simulink model "GNC_exp_simulink_vision"  (R2018a)
settings: Solver=FixedStepAuto  StartTime=0.0  StopTime=50  FixedStep=0.2  MaxStep=0.5  MinStep=0.3  RelTol=10  AbsTol=10
values from neighbouring files (symbols this model uses):
  flightplan = [0,2*dist,height,deg2rad(180) ... (first row only)    [initialize_exp.m]    (also in initialize_race_flighttest.m; initialize_race_realtime.m = [dist,0,height,deg2rad(090))
  FOV = 1.05    [initialize_exp.m]    (also in initialize_race_flighttest.m; initialize_race_realtime.m)
  g = 9.81    [initialize_exp.m]    (also in initialize_race_flighttest.m; initialize_race_realtime.m)
  gate_size = 1.4    [initialize_exp.m]    (also in initialize_race_flighttest.m; initialize_race_realtime.m)
  max_rot_Z = max_vel*(60)*pi/180    (= 0.523598775598)    [initialize_exp.m]    (also in initialize_race_flighttest.m; initialize_race_realtime.m = 1.57079632679)
  max_theta_X = 75*pi/180    (= 1.308996939)    [initialize_exp.m]    (also in initialize_race_flighttest.m; initialize_race_realtime.m)
  max_theta_Y = 75*pi/180    (= 1.308996939)    [initialize_exp.m]    (also in initialize_race_flighttest.m; initialize_race_realtime.m)
  max_v_Z = 2*max_vel    (= 1)    [initialize_exp.m]    (also in initialize_race_flighttest.m; initialize_race_realtime.m = 3)
  max_vel = 0.5    [initialize_exp.m]    (also in initialize_race_flighttest.m; initialize_race_realtime.m = 1.5)
  spline_init = [P0;P1;P2;P3]    [initialize_exp.m]    (also in initialize_race_flighttest.m; initialize_race_realtime.m)
undefined symbols (not defined in the file or in its folder): eul, gray, HFOV, pos, Rec, resolution, SDTV, two_std_dev_init, two_std_dev_thres, vel, VFOV
libraries: visiontextngfix x5, simulink x3, sharedtransform x3, aerolibutil x2, visionconversions x2, visionanalysis x1, visionstatistics x1, visiontransforms x1
(part 3 of 3)

== matlab function GNC_exp_simulink_vision/Guidance/filter_WP_moving_av ==
  data: WP_list_out output; WP_idx_out output; WP_list_in input; WP_idx_in input; dist_old_raw input; WP_current_pos input; WP_current_eul input; WP_std_dev_out output; WP_est_out output; WP_P_mat_out output; two_init_std_dev input; WP_list_const input; WP_est_in input; WP_P_mat_in input
function [WP_list_out, WP_idx_out, WP_std_dev_out, WP_est_out, WP_P_mat_out] = ...
    filter_WP(WP_list_in, WP_idx_in, dist_old_raw, WP_current_pos, WP_current_eul, two_init_std_dev, WP_list_const, WP_est_in, WP_P_mat_in)
    
    mean_var = diag(0.1*ones(4,1));
    
    % catch script start
    if isequal(WP_P_mat_in,ones(4,4))
        WP_P_mat_in = diag((two_init_std_dev/2).^2);
        WP_est_in = WP_list_const(1,:)';
    end
    
    % catch state transition
    WP_idx_out = WP_idx_in;
    if dist_old_raw > 1
        disp('new state')
        WP_idx_out = WP_idx_out+1;
        if WP_idx_out == size(WP_list_in,1)
            WP_idx_out = 0;
        end
        WP_est_in = WP_list_const(WP_idx_out+1,:)';
        %WP_current_gate_in = WP_list_const(WP_idx_out+1,:)';
        WP_P_mat_in = diag((two_init_std_dev/2).^2);
    end
    WP_current_gate = WP_list_const(WP_idx_out+1,:)';
    WP_list_out = WP_list_in;
    
    WP_P_mat_out = WP_P_mat_in;
    WP_std_dev_out = sqrt(diag(WP_P_mat_out));
    
    WP_est_out = WP_est_in;
    
   
    if WP_current_eul(1) > WP_current_gate(4) + pi/2
        euler_used = WP_current_eul(1)-pi;
    elseif WP_current_eul(1) < WP_current_gate(4)-pi/2
        euler_used = WP_current_eul(1)+pi;
    else
        euler_used = WP_current_eul(1);
    end
        
    % check if there is gate information
    if isequal(WP_current_eul, zeros(1,3)) || isequal(WP_current_eul, zeros(3,1))
        % no gate info
        %         disp('gate_global - no corners')
        
    else

        
        if (norm(WP_current_pos(1:2) - WP_current_gate(1:2)) > 2.0) ||...
                WP_current_pos(1) - WP_est_in(1) > 3*sqrt(WP_P_mat_in(1,1)) || ...
                WP_current_pos(2) - WP_est_in(2) > 3*sqrt(WP_P_mat_in(2,2))
                %sqrt(WP_P_mat_in(4,4)) < 0.1 && ...
                %sqrt(WP_P_mat_in(3,3)) < 0.1 && ...
                %sqrt(WP_P_mat_in(2,2)) < 0.1 && ...
                %sqrt(WP_P_mat_in(1,1)) < 0.1) || WP_idx_out ~= WP_idx_out
            %WP_current = [WP_current_pos; WP_current_eul(1)];
            
            %K_gain = WP_P_mat_in*inv(WP_P_mat_in + mean_var);
            
            WP_est_out = WP_est_in;% + K_gain*(WP_current - WP_est_in);
            WP_P_mat_out = WP_P_mat_in;
            
            WP_list_out(WP_idx_out+1,:) = WP_est_out';
            WP_std_dev_out = sqrt(diag(WP_P_mat_out));
            
        else
            
            WP_current = [WP_current_pos; euler_used];
            
            K_gain = WP_P_mat_in*inv(WP_P_mat_in + mean_var);
            
            delta = WP_current-WP_est_in;
            delta(4) = WP_current(4)-WP_est_in(4); %angle_add(WP_current(4),-WP_est_in(4));
            
            WP_est_out(1:3) = WP_est_in(1:3) + K_gain(1:3,:)*(delta);
            WP_est_out(4) = WP_est_in(4) + K_gain(4,:)*delta; %angle_add(WP_est_in(4),K_gain(4,:)*delta);
            WP_P_mat_out = (eye(4) - K_gain)*WP_P_mat_in;
            
            WP_list_out(WP_idx_out+1,:) = WP_est_out';
            WP_std_dev_out = sqrt(diag(WP_P_mat_out));
        end

%         lambda = 0.1;
%         
%         WP_average = WP_list_out(WP_idx_out+1,:)';
%         
%        
%         delta = WP_current-WP_average;
%         delta(4) = angle_add(WP_current(4),-WP_average(4));
%         std = abs(delta) ./ sqrt(WP_std_dev_out);
%     
%         alpha = lambda.^(2*std);
%         alpha = min(alpha, lambda);
% %         alpha = max(alpha, 0.001);
%         WP_average(1:3) = WP_average(1:3) + alpha(1:3).*delta(1:3);
%         WP_average(4) = angle_add(WP_average(4),alpha(4)*delta(4));
%         
%         WP_std_dev_out = sqrt((1-alpha).*(WP_std_dev_out.^2+alpha.*delta.*delta));
% 
%         WP_list_out(WP_idx_out+1,:) = WP_average;
        
    end
end

function sum = angle_add(a1,a2)
    sum = atan2(sin(a1+a2),cos(a1+a2));
end



% 
%         if norm(WP_current_pos' - WP_average_pos) < 0.7
%             WP_average_pos = alpha*WP_current_pos' + (1-alpha)*WP_average_pos;
%             WP_current_hdg = WP_current_ori(1);
%             WP_average_hdg = atan2(alpha*sin(WP_current_hdg) + (1-alpha)*sin(WP_average_hdg), ...
%                 alpha*cos(WP_current_hdg) + (1-alpha)*cos(WP_average_hdg));
%             WP_average = [WP_average_pos, WP_average_hdg];
%             WP_list_out(state0_out+1,:) = WP_average;
%         end

== matlab function GNC_exp_simulink_vision/Vision System/gate_global ==
  data: tVec input; rMat input; drone_pos input; drone_ori input; gate_pos_global output; gate_eul_global output
function [gate_pos_global, gate_eul_global]  = gate_global(tVec, rMat, drone_pos, drone_ori)

    gate_pos_global = zeros(3,1);
    gate_eul_global = zeros(3,1);
%     drone_rotm = axang2rotm(drone_ori');
%     gate_pos_local = quatrotate(drone_q,gate_pos_cam);
%     gate_pos_local = drone_rotm * gate_pos_cam';
%     gate_pos_global = gate_pos_local + drone_pos';
%     gate_pos_global = gate_pos_local;

if isequal(tVec,zeros(1,3))
%     disp('gate_global - no corners')
    return
end
    
    %% drone pos
    drone_pos;
    
    %% drone orientation
    dRg = eul2rotm([drone_ori(3),drone_ori(2),drone_ori(1)]);
    
    %% convert gate pos
    % tVec = right down front, drone was front left up
    dRc = eul2rotm([pi/2,-pi/2,0],'ZYX');
    cRd = dRc^-1;
    cRg = dRg*cRd;
    rel= cRg*tVec';
    gate_pos_global = drone_pos + rel;
    
    % rel = -dRs*tvec';
    % gate_pos_global = drone_pos + rel';
    
    %% convert gate orientation
    rot = squeeze(rMat);
    extra = eul2rotm([0,pi/2,0],'ZYX');
    gate_rot = dRg*cRd*rot^-1*extra;
    gate_eul_global = rotm2eul(gate_rot)';
%     
%     wRc = rMat;
%     one_more = 1;%eul2rotm([pi,0,-pi/2]);
%     another_one = 1;%eul2rotm([pi/2,0,0]);
%     wRs = another_one*one_more*cRg*wRc;
%     
%     gate_ori_global = (rotm2eul(wRs))';

%       rot = rMat*cRg^-1;
%       gate_yaw=rotm2eul(rot);
    
end
